simulink model "PID_control"  (R2020b)
settings: Solver=VariableStepAuto  StartTime=0.0  StopTime=10.0  FixedStep=0.0000002  RelTol=1e-3
undefined symbols (not defined in the file or in its folder): Kd, Ki, Kp
settings Model: DataDictionary=DC_Motor_data.sldd  Creator=JAGRUTI SHINDE  LastModifiedBy=JAGRUTI SHINDE
settings DataIOCC: SaveOutput=off  SaveTime=off

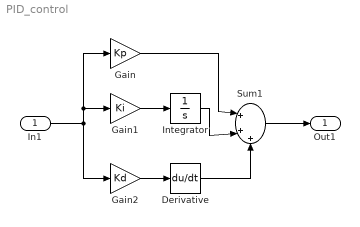
== system PID_control ==
  In1 : Inport  OutDataTypeStr=double  PortDimensions=1  SampleTime=0
  Derivative : Derivative
  Gain : Gain  Gain=Kp
  Gain1 : Gain  Gain=Ki
  Gain2 : Gain  Gain=Kd
  Integrator : Integrator
  Sum1 : Sum  Inputs=|+++
  Out1 : Outport  OutDataTypeStr=double  PortDimensions=1  SampleTime=0
  wires:
  Gain/1 -> Sum1/1
  In1/1 -> Gain2/1, Gain/1, Gain1/1
  Integrator/1 -> Sum1/2
  Derivative/1 -> Sum1/3
  Gain2/1 -> Derivative/1
  Sum1/1 -> Out1/1
  Gain1/1 -> Integrator/1
